simulink model "SG_periodicWalk"  (R2022a)
settings: Solver=ode4  StartTime=0.0  StopTime=20  FixedStep=1/(communication_rate*2)  MaxStep=0.001  RelTol=1e-3  AbsTol=1e-3  EnableMultiTasking=on
values from neighbouring files (symbols this model uses):
  dphi_IC = Gains.dphi_IC    [Controller.m]
  dr_IC = Gains.dr_IC    [Controller.m]
  Kd_phi_IC = Gains.Kd_phi_IC    [Controller.m]
  Kd_r_IC = Gains.Kd_r_IC    [Controller.m]
  Kp_phi_IC = Gains.Kp_phi_IC    [Controller.m]
  Kp_r_IC = Gains.Kp_r_IC    [Controller.m]
  phi_IC = Gains.phi_IC    [Controller.m]
  r_IC = Gains.r_IC    [Controller.m]
undefined symbols (not defined in the file or in its folder): communication_rate, HS, IO291, Kd, Kp, match_leg_gains
libraries: speedgoatlib_IO691 x11, canmsglib x10, simulink x4, aru_toolbox x3, speedgoatlib_IO291 x2
(part 2 of 2)

== matlab function SG_periodicWalk/SubsysteM3/Read Block/Motor 3 Read - THETA3/MATLAB Function2 ==
  data: pos_h input; final_pos output; pos_l input; vel_h input; vel_l input; i_h input; i_l input; final_vel output; final_i output
function [final_pos,final_vel,final_i] = fcn(pos_h,pos_l,vel_h,vel_l,i_h,i_l)
% ------------------------------------
max_pos = 12.5;
min_pos = -12.5;
span_pos = max_pos - min_pos;
offset_pos = max_pos;

pos = bitshift(pos_h,8);
combined_pos = bitor(pos,pos_l);

range_pos = ((combined_pos*span_pos)/(2^16-1))-offset_pos;

final_pos = (range_pos*4*pi)/12.5;
% ------------------------------------
max_vel = 50;
min_vel = -50;
span_vel = max_vel - min_vel;
offset_vel = max_vel;
vel = bitshift(vel_h,4);
combined_vel = bitor(vel,vel_l);

final_vel = ((combined_vel*span_vel)/(2^12-1))-offset_vel;

% ------------------------------------
max_i = 65;
min_i = -65;
span_i = max_i - min_i;
offset_i = max_i;
i = bitshift(i_h,8);
combined_i = bitor(i,i_l);

final_i = ((combined_i*span_i)/(2^12-1))-offset_i;
end

== matlab function SG_periodicWalk/SubsysteM3/Write Block/MATLAB Function7 ==
  data: motorCMD input; q output; w output; Kp output; Kd output; tff output
function [q,w,Kp,Kd,tff] = cmd(motorCMD)

    q = motorCMD.q;
    w = motorCMD.w;
    Kp = motorCMD.Kp;
    Kd = motorCMD.Kd;
    tff = motorCMD.tff;

end

== matlab function SG_periodicWalk/CMD_M23/M43 ==
  settings: updateMethod=DISCRETE
  data: Gains input; match_leg_gains input; tau1 output; tau2 output; M2_State input; activateTrajectories output; M3_State input
function [tau1,tau2,activateTrajectories]  = RController(Gains,match_leg_gains,M2_State,M3_State)

    if match_leg_gains == -1
        theta_ML = M2_State.q;
        dtheta_ML = M2_State.w;
        theta_MR = M3_State.q;
        dtheta_MR = M3_State.w;
    else
        theta_ML = M3_State.q;
        dtheta_ML = M3_State.w;
        theta_MR = M2_State.q;
        dtheta_MR = M2_State.w;
    end

%     tau1 = match_leg_gains*M2_State.t;
%     tau2 = match_leg_gains*M3_State.t;

    [B,activateTrajectories] = Controller(Gains,theta_ML,theta_MR,dtheta_ML,dtheta_MR);
    tau1 = B(1);
    tau2 = B(2);
    
   
end

== matlab function SG_periodicWalk/SubsysteM3/Write Block/MATLAB Function3 ==
  data: p_des input; P8H output; v_des input; kp input; kd input; t_ff input; P8L output; V8H output; M2L output; KP4H output; KP8L output; KD8H output; KD4L output; T4H output; T8L output
function [P8H,P8L,V8H,M2L,KP4H,KP8L,KD8H,KD4L,T4H,T8L] = AK1090(p_des, v_des, kp, kd, t_ff)
    % Coppied from AK70-10 manual
    % NB: CONSTANTS FOR AK70-10
    p_min = -12.5; % rad
    p_max = +12.5; % rad
    v_min = -50.0; % rad/s
    v_max = +50.0; % rad/s
    t_min = -65.0; % Nm
    t_max = +65.0; % Nm
    kp_min = 0;
    kp_max = 500;
    kd_min = 0;
    kd_max = 5;
    
    % bound inputs
    p_des = min([max([p_min,p_des]),p_max]);
    v_des = min([max([v_min,v_des]),v_max]);
    kp = min([max([kp_min,kp]),kp_max]);
    kd = min([max([kd_min,kd]),kd_max]);
    t_ff = min([max([t_min,t_ff]),t_max]);
    
    % convert floats to unsigned integers
    p_int = float_to_uint(p_des, p_min, p_max, 16);
    v_int = float_to_uint(v_des, v_min, v_max, 12);
    kp_int = float_to_uint(kp, kp_min, kp_max, 12);
    kd_int = float_to_uint(kd, kd_min, kd_max, 12);
    t_int = float_to_uint(t_ff, t_min, t_max, 12);
    
    % break up for CAN frame 
    P8H = bitshift(p_int, -8); % 8 higher bits
    P8L = bitand(p_int, 0xFF); % 8 lower bits
    V8H = bitshift(v_int, -4); % 8 higher bits
    M2L = bitand(v_int, 0xF); % 4 lower bits
    KP4H = bitshift(kp_int, -8); % 4 higher bits
    KP8L = bitand(kp_int, 0xFF); % 8 lower bits
    KD8H = bitshift(kd_int, -4); % 8 higher bits
    KD4L = bitand(kd_int, 0xF); % 4 lower bits
    T4H = bitshift(t_int, -8); % 4 higher bits
    T8L = bitand(t_int, 0xFF); % 8 lower bits
    
    % Converts a float to an unsigned int, given range and number of bits
    function x_int = float_to_uint(x, x_min, x_max, n_bits)
        span = x_max - x_min;
        min([max([x_min,x]),x_max])
        x_int = ((x - x_min)*(bitshift(1, n_bits) / span));
    end
end
%final_values = desired_pos,desired_vel,desired_kp,desired_kd,desired_tau;

== matlab function SG_periodicWalk/CMD_M23/MATLAB Function ==
  data: Gains input; pos_M2_des input; pos_M3_des input; vel_M2_des input; vel_M3_des input; tau_M2_des input; tau_M3_des input; tau1 input; tau2 input; pos_M2 output; vel_M2 output; Kp_M2 output; Kd_M2 output; activateTrajectories input; tau_M2 output; pos_M3 output; vel_M3 output; Kp_M3 output; Kd_M3 output; tau_M3 output
function [pos_M2,vel_M2,Kp_M2,Kd_M2,tau_M2,pos_M3,vel_M3,Kp_M3,Kd_M3,tau_M3] = dataSelection(Gains,pos_M2_des,pos_M3_des,vel_M2_des,vel_M3_des,tau_M2_des,tau_M3_des,tau1,tau2,activateTrajectories)

    if activateTrajectories == 1
        pos_M2 = pos_M2_des;
        pos_M3 = pos_M3_des;
        vel_M2 = vel_M2_des;
        vel_M3 = vel_M3_des;
        tau_M2 = tau_M2_des;
        tau_M3 = tau_M3_des;
        Kp_M2 = Gains.Kp;
        Kd_M2 = Gains.Kd;
        Kp_M3 = Gains.Kp;
        Kd_M3 = Gains.Kd;
    else
        pos_M2 = 0;
        pos_M3 = 0;
        vel_M2 = 0;
        vel_M3 = 0;
        tau_M2 = tau1;
        tau_M3 = tau2;
        Kp_M2 = 0;
        Kd_M2 = 0;
        Kp_M3 = 0;
        Kd_M3 = 0;
    end
end

== matlab function SG_periodicWalk/CMD_M14/M43 ==
  settings: updateMethod=DISCRETE
  data: Gains input; tau1 output; tau2 output; M1_State input; activateTrajectories output; M4_State input
function [tau1,tau2,activateTrajectories]  = RController(Gains,M1_State,M4_State)
    theta_ML = M1_State.q;
    theta_MR = M4_State.q;
    dtheta_ML = M1_State.w;
    dtheta_MR = M4_State.w;
    [B,activateTrajectories] = Controller(Gains,theta_ML,theta_MR,dtheta_ML,dtheta_MR);
    tau1 = B(1);
    tau2 = B(2);
   
end

== matlab function SG_periodicWalk/CMD_M14/MATLAB Function ==
  data: Gains input; pos_M1_des input; pos_M4_des input; vel_M1_des input; vel_M4_des input; tau_M1_des input; tau_M4_des input; tau1 input; tau2 input; pos_M1 output; vel_M1 output; Kp_M1 output; Kd_M1 output; activateTrajectories input; tau_M1 output; pos_M4 output; vel_M4 output; Kp_M4 output; Kd_M4 output; tau_M4 output
function [pos_M1,vel_M1,Kp_M1,Kd_M1,tau_M1,pos_M4,vel_M4,Kp_M4,Kd_M4,tau_M4] = dataSelection(Gains,pos_M1_des,pos_M4_des,vel_M1_des,vel_M4_des,tau_M1_des,tau_M4_des,tau1,tau2,activateTrajectories)

    if activateTrajectories == 1
        pos_M1 = pos_M1_des;
        pos_M4 = pos_M4_des;
        vel_M1 = vel_M1_des;
        vel_M4 = vel_M4_des;
        tau_M1 = tau_M1_des;
        tau_M4 = tau_M4_des;
        Kp_M1 = Gains.Kp;
        Kd_M1 = Gains.Kd;
        Kp_M4 = Gains.Kp;
        Kd_M4 = Gains.Kd;
    else
        pos_M1 = 0;
        pos_M4 = 0;
        vel_M1 = 0;
        vel_M4 = 0;
        tau_M1 = tau1;
        tau_M4 = tau2;
        Kp_M1 = 0;
        Kd_M1 = 0;
        Kp_M4 = 0;
        Kd_M4 = 0;
    end
end

== matlab function SG_periodicWalk/SubsysteM3/MATLAB Function ==
  data: x input; y input; state output Bus: BodyState; r input; dx input; dy input; dr input; ddx input; ddy input; ddr input
function state  = boom_state(x,y,r,dx,dy,dr,ddx,ddy,ddr)
state.x = x;
state.dx = dx;
state.ddx = ddx;

state.y = y;
state.dy = dy;
state.ddy = ddy;

state.r = r;
state.dr = dr;
end

== matlab function SG_periodicWalk/SubsysteM3/Write Block/MATLAB Function2 ==
  data: p_des input; P8H output; v_des input; kp input; kd input; t_ff input; P8L output; V8H output; M2L output; KP4H output; KP8L output; KD8H output; KD4L output; T4H output; T8L output
function [P8H,P8L,V8H,M2L,KP4H,KP8L,KD8H,KD4L,T4H,T8L] = AK1090(p_des, v_des, kp, kd, t_ff)
    % Coppied from AK70-10 manual
    % NB: CONSTANTS FOR AK70-10
    p_min = -12.5; % rad
    p_max = +12.5; % rad
    v_min = -50.0; % rad/s
    v_max = +50.0; % rad/s
    t_min = -65.0; % Nm
    t_max = +65.0; % Nm
    kp_min = 0;
    kp_max = 500;
    kd_min = 0;
    kd_max = 5;
    
    % bound inputs
    p_des = min([max([p_min,p_des]),p_max]);
    v_des = min([max([v_min,v_des]),v_max]);
    kp = min([max([kp_min,kp]),kp_max]);
    kd = min([max([kd_min,kd]),kd_max]);
    t_ff = min([max([t_min,t_ff]),t_max]);
    
    % convert floats to unsigned integers
    p_int = float_to_uint(p_des, p_min, p_max, 16);
    v_int = float_to_uint(v_des, v_min, v_max, 12);
    kp_int = float_to_uint(kp, kp_min, kp_max, 12);
    kd_int = float_to_uint(kd, kd_min, kd_max, 12);
    t_int = float_to_uint(t_ff, t_min, t_max, 12);
    
    % break up for CAN frame 
    P8H = bitshift(p_int, -8); % 8 higher bits
    P8L = bitand(p_int, 0xFF); % 8 lower bits
    V8H = bitshift(v_int, -4); % 8 higher bits
    M2L = bitand(v_int, 0xF); % 4 lower bits
    KP4H = bitshift(kp_int, -8); % 4 higher bits
    KP8L = bitand(kp_int, 0xFF); % 8 lower bits
    KD8H = bitshift(kd_int, -4); % 8 higher bits
    KD4L = bitand(kd_int, 0xF); % 4 lower bits
    T4H = bitshift(t_int, -8); % 4 higher bits
    T8L = bitand(t_int, 0xFF); % 8 lower bits
    
    % Converts a float to an unsigned int, given range and number of bits
    function x_int = float_to_uint(x, x_min, x_max, n_bits)
        span = x_max - x_min;
        min([max([x_min,x]),x_max])
        x_int = ((x - x_min)*(bitshift(1, n_bits) / span));
    end
end
%final_values = desired_pos,desired_vel,desired_kp,desired_kd,desired_tau;

== matlab function SG_periodicWalk/SubsysteM3/Write Block/MATLAB Function4 ==
  data: motorCMD input; q output; w output; Kp output; Kd output; tff output
function [q,w,Kp,Kd,tff] = cmd(motorCMD)

    q = motorCMD.q;
    w = motorCMD.w;
    Kp = motorCMD.Kp;
    Kd = motorCMD.Kd;
    tff = motorCMD.tff;

end

== matlab function SG_periodicWalk/SubsysteM3/Read Block/CAN Read Loop - Port 3/MATLAB Function1 ==
  data: pos_h input; final_pos output; pos_l input; vel_h input; vel_l input; i_h input; i_l input; final_vel output; final_i output
function [final_pos,final_vel,final_i] = fcn(pos_h,pos_l,vel_h,vel_l,i_h,i_l)
% ------------------------------------
max_pos = 12.5;
min_pos = -12.5;
span_pos = max_pos - min_pos;
offset_pos = max_pos;

pos = bitshift(pos_h,8);
combined_pos = bitor(pos,pos_l);

range_pos = ((combined_pos*span_pos)/(2^16-1))-offset_pos;

final_pos = (range_pos*4*pi)/12.5;
% ------------------------------------
max_vel = 50;
min_vel = -50;
span_vel = max_vel - min_vel;
offset_vel = max_vel;
vel = bitshift(vel_h,4);
combined_vel = bitor(vel,vel_l);

final_vel = ((combined_vel*span_vel)/(2^12-1))-offset_vel;

% ------------------------------------
max_i = 65;
min_i = -65;
span_i = max_i - min_i;
offset_i = max_i;
i = bitshift(i_h,8);
combined_i = bitor(i,i_l);

final_i = ((combined_i*span_i)/(2^12-1))-offset_i;
end

== matlab function SG_periodicWalk/SubsysteM3/Write Block/MATLAB Function1 ==
  data: p_des input; P8H output; v_des input; kp input; kd input; t_ff input; P8L output; V8H output; M2L output; KP4H output; KP8L output; KD8H output; KD4L output; T4H output; T8L output
function [P8H,P8L,V8H,M2L,KP4H,KP8L,KD8H,KD4L,T4H,T8L] = AK1090(p_des, v_des, kp, kd, t_ff)
    % Coppied from AK70-10 manual
    % NB: CONSTANTS FOR AK70-10
    p_min = -12.5; % rad
    p_max = +12.5; % rad
    v_min = -50.0; % rad/s
    v_max = +50.0; % rad/s
    t_min = -65.0; % Nm
    t_max = +65.0; % Nm
    kp_min = 0;
    kp_max = 500;
    kd_min = 0;
    kd_max = 5;
    
    % bound inputs
    p_des = min([max([p_min,p_des]),p_max]);
    v_des = min([max([v_min,v_des]),v_max]);
    kp = min([max([kp_min,kp]),kp_max]);
    kd = min([max([kd_min,kd]),kd_max]);
    t_ff = min([max([t_min,t_ff]),t_max]);
    
    % convert floats to unsigned integers
    p_int = float_to_uint(p_des, p_min, p_max, 16);
    v_int = float_to_uint(v_des, v_min, v_max, 12);
    kp_int = float_to_uint(kp, kp_min, kp_max, 12);
    kd_int = float_to_uint(kd, kd_min, kd_max, 12);
    t_int = float_to_uint(t_ff, t_min, t_max, 12);
    
    % break up for CAN frame 
    P8H = bitshift(p_int, -8); % 8 higher bits
    P8L = bitand(p_int, 0xFF); % 8 lower bits
    V8H = bitshift(v_int, -4); % 8 higher bits
    M2L = bitand(v_int, 0xF); % 4 lower bits
    KP4H = bitshift(kp_int, -8); % 4 higher bits
    KP8L = bitand(kp_int, 0xFF); % 8 lower bits
    KD8H = bitshift(kd_int, -4); % 8 higher bits
    KD4L = bitand(kd_int, 0xF); % 4 lower bits
    T4H = bitshift(t_int, -8); % 4 higher bits
    T8L = bitand(t_int, 0xFF); % 8 lower bits
    
    % Converts a float to an unsigned int, given range and number of bits
    function x_int = float_to_uint(x, x_min, x_max, n_bits)
        span = x_max - x_min;
        min([max([x_min,x]),x_max])
        x_int = ((x - x_min)*(bitshift(1, n_bits) / span));
    end
end
%final_values = desired_pos,desired_vel,desired_kp,desired_kd,desired_tau;
